simulink model "ACC"  (Simulink 7.5)
settings: Solver=ode45  StartTime=0.0  StopTime=inf  RelTol=1e-3
libraries: CarMaker4SL x24, simulink x2
(part 2 of 2)

== system ACC/CarMaker/Vehicle/CarAndTrailer/Trailer/CreateBus Car.Hitch.FrcTrq ==
  In1 : Inport  OutDataType=sfix(16)  OutScaling=2^0
  Bus Creator7 : BusCreator  Inputs=6
  Demux7 : Demux  Outputs=6
  Car.Hitch.FrcTrq : Outport  OutDataType=sfix(16)  OutScaling=2^0
  wires:
  Demux7/1 -> Bus Creator7/1  "Car Hitch Frc2Car x"
  Demux7/2 -> Bus Creator7/2  "Car Hitch Frc2Car y"
  Demux7/3 -> Bus Creator7/3  "Car Hitch Frc2Car z"
  Demux7/4 -> Bus Creator7/4  "Car Hitch Trq2Car x"
  Demux7/5 -> Bus Creator7/5  "Car Hitch Trq2Car y"
  Demux7/6 -> Bus Creator7/6  "Car Hitch Trq2Car z"
  Bus Creator7/1 -> Car.Hitch.FrcTrq/1
  In1/1 -> Demux7/1

== system ACC/CarMaker/Vehicle/CarAndTrailer/Trailer/CreateBus Vhcl.Motion ==
  In1 : Inport  OutDataType=sfix(16)  OutScaling=2^0
  Demux1 : Demux  Outputs=16
  Mux1 : Mux  Inputs=16
  Out1 : Outport  OutDataType=sfix(16)  OutScaling=2^0
  wires:
  Mux1/1 -> Out1/1
  In1/1 -> Demux1/1
  Demux1/16 -> Mux1/16  "Vhcl YawAcc"
  Demux1/15 -> Mux1/15  "Vhcl YawRate"
  Demux1/14 -> Mux1/14  "Vhcl Yaw"
  Demux1/13 -> Mux1/13  "Vhcl PitchAcc"
  Demux1/12 -> Mux1/12  "Vhcl PitchVel"
  Demux1/11 -> Mux1/11  "Vhcl Pitch"
  Demux1/10 -> Mux1/10  "Vhcl RollAcc"
  Demux1/9 -> Mux1/9  "Vhcl RollVel"
  Demux1/8 -> Mux1/8  "Vhcl Roll"
  Demux1/7 -> Mux1/7  "Vhcl Hitch_Pos z"
  Demux1/6 -> Mux1/6  "Vhcl Hitch_Pos y"
  Demux1/5 -> Mux1/5  "Vhcl Hitch_Pos x"
  Demux1/4 -> Mux1/4  "Vhcl sRoadAero"
  Demux1/3 -> Mux1/3  "Vhcl sRoad"
  Demux1/2 -> Mux1/2  "Vhcl Distance"
  Demux1/1 -> Mux1/1  "Vhcl v"

== system ACC/CarMaker/Vehicle/CarAndTrailer/Trailer/CreateBus Vhcl.PoI ==
  In1 : Inport  OutDataType=sfix(16)  OutScaling=2^0
  Bus Creator3 : BusCreator  Inputs=18
  Demux3 : Demux  Outputs=18
  Out1 : Outport  OutDataType=sfix(16)  OutScaling=2^0
  wires:
  Demux3/1 -> Bus Creator3/1  "Vhcl PoI_Pos x"
  Bus Creator3/1 -> Out1/1
  In1/1 -> Demux3/1
  Demux3/2 -> Bus Creator3/2  "Vhcl PoI_Pos y"
  Demux3/3 -> Bus Creator3/3  "Vhcl PoI_Pos z"
  Demux3/4 -> Bus Creator3/4  "Vhcl PoI_Vel x"
  Demux3/5 -> Bus Creator3/5  "Vhcl PoI_Vel y"
  Demux3/6 -> Bus Creator3/6  "Vhcl PoI_Vel z"
  Demux3/7 -> Bus Creator3/7  "Vhcl PoI_Acc x"
  Demux3/8 -> Bus Creator3/8  "Vhcl PoI_Acc y"
  Demux3/9 -> Bus Creator3/9  "Vhcl PoI_Acc z"
  Demux3/10 -> Bus Creator3/10  "Vhcl PoI_Vel_1 x"
  Demux3/11 -> Bus Creator3/11  "Vhcl PoI_Vel_1 y"
  Demux3/12 -> Bus Creator3/12  "Vhcl PoI_Vel_1 z"
  Demux3/13 -> Bus Creator3/13  "Vhcl PoI_Acc_1 x"
  Demux3/14 -> Bus Creator3/14  "Vhcl PoI_Acc_1 y"
  Demux3/15 -> Bus Creator3/15  "Vhcl PoI_Acc_1 z"
  Demux3/16 -> Bus Creator3/16  "Vhcl PoI_GCS Long"
  Demux3/17 -> Bus Creator3/17  "Vhcl PoI_GCS Lat"
  Demux3/18 -> Bus Creator3/18  "Vhcl PoI_GCS Elev"

== system ACC/CarMaker/Vehicle/CarAndTrailer/Trailer/CreateBus Vhcl.Steering ==
  In1 : Inport  OutDataType=sfix(16)  OutScaling=2^0
  Bus Creator3 : BusCreator
  Demux : Demux
  Out1 : Outport  OutDataType=sfix(16)  OutScaling=2^0
  wires:
  In1/1 -> Demux/1
  Demux/4 -> Bus Creator3/4  "Vhcl Steering Trq"
  Demux/2 -> Bus Creator3/2  "Vhcl Steering AngVel"
  Demux/3 -> Bus Creator3/3  "Vhcl Steering AngAcc"
  Demux/1 -> Bus Creator3/1  "Vhcl Steering Ang"
  Bus Creator3/1 -> Out1/1

== system ACC/CarMaker/Vehicle/CarAndTrailer/Trailer/CreateBus Vhcl.Wheel.FL ==
  In1 : Inport  OutDataType=sfix(16)  OutScaling=2^0
  Bus Creator3 : BusCreator  Inputs=14
  Demux3 : Demux  Outputs=14
  Out1 : Outport  OutDataType=sfix(16)  OutScaling=2^0
  wires:
  Demux3/1 -> Bus Creator3/1  "Vhcl Wheel FL t x"
  Bus Creator3/1 -> Out1/1
  In1/1 -> Demux3/1
  Demux3/2 -> Bus Creator3/2  "Vhcl Wheel FL t y"
  Demux3/3 -> Bus Creator3/3  "Vhcl Wheel FL t z"
  Demux3/4 -> Bus Creator3/4  "Vhcl Wheel FL r_zxy x"
  Demux3/5 -> Bus Creator3/5  "Vhcl Wheel FL r_zxy y"
  Demux3/6 -> Bus Creator3/6  "Vhcl Wheel FL r_zxy z"
  Demux3/7 -> Bus Creator3/7  "Vhcl Wheel FL Fx"
  Demux3/8 -> Bus Creator3/8  "Vhcl Wheel FL Fy"
  Demux3/9 -> Bus Creator3/9  "Vhcl Wheel FL Fz"
  Demux3/10 -> Bus Creator3/10  "Vhcl Wheel FL vBelt"
  Demux3/11 -> Bus Creator3/11  "Vhcl Wheel FL LongSlip"
  Demux3/12 -> Bus Creator3/12  "Vhcl Wheel FL SideSlip"
  Demux3/13 -> Bus Creator3/13  "Vhcl Wheel FL Trq_T2W"
  Demux3/14 -> Bus Creator3/14  "Vhcl Wheel FL Trq_WhlBearing"

== system ACC/CarMaker/Vehicle/CarAndTrailer/Trailer/CreateBus Vhcl.Wheel.FR ==
  In1 : Inport  OutDataType=sfix(16)  OutScaling=2^0
  Bus Creator3 : BusCreator  Inputs=14
  Demux3 : Demux  Outputs=14
  Out1 : Outport  OutDataType=sfix(16)  OutScaling=2^0
  wires:
  Demux3/1 -> Bus Creator3/1  "Vhcl Wheel FR t x"
  Bus Creator3/1 -> Out1/1
  In1/1 -> Demux3/1
  Demux3/2 -> Bus Creator3/2  "Vhcl Wheel FR t y"
  Demux3/3 -> Bus Creator3/3  "Vhcl Wheel FR t z"
  Demux3/4 -> Bus Creator3/4  "Vhcl Wheel FR r_zxy x"
  Demux3/5 -> Bus Creator3/5  "Vhcl Wheel FR r_zxy y"
  Demux3/6 -> Bus Creator3/6  "Vhcl Wheel FR r_zxy z"
  Demux3/7 -> Bus Creator3/7  "Vhcl Wheel FR Fx"
  Demux3/8 -> Bus Creator3/8  "Vhcl Wheel FR Fy"
  Demux3/9 -> Bus Creator3/9  "Vhcl Wheel FR Fz"
  Demux3/10 -> Bus Creator3/10  "Vhcl Wheel FR vBelt"
  Demux3/11 -> Bus Creator3/11  "Vhcl Wheel FR LongSlip"
  Demux3/12 -> Bus Creator3/12  "Vhcl Wheel FR SideSlip"
  Demux3/13 -> Bus Creator3/13  "Vhcl Wheel FR Trq_T2W"
  Demux3/14 -> Bus Creator3/14  "Vhcl Wheel FR Trq_WhlBearing"

== system ACC/CarMaker/Vehicle/CarAndTrailer/Trailer/CreateBus Vhcl.Wheel.RL ==
  In1 : Inport  OutDataType=sfix(16)  OutScaling=2^0
  Bus Creator3 : BusCreator  Inputs=14
  Demux3 : Demux  Outputs=14
  Out1 : Outport  OutDataType=sfix(16)  OutScaling=2^0
  wires:
  Demux3/1 -> Bus Creator3/1  "Vhcl Wheel RL t x"
  Bus Creator3/1 -> Out1/1
  In1/1 -> Demux3/1
  Demux3/2 -> Bus Creator3/2  "Vhcl Wheel RL t y"
  Demux3/3 -> Bus Creator3/3  "Vhcl Wheel RL t z"
  Demux3/4 -> Bus Creator3/4  "Vhcl Wheel RL r_zxy x"
  Demux3/5 -> Bus Creator3/5  "Vhcl Wheel RL r_zxy y"
  Demux3/6 -> Bus Creator3/6  "Vhcl Wheel RL r_zxy z"
  Demux3/7 -> Bus Creator3/7  "Vhcl Wheel RL Fx"
  Demux3/8 -> Bus Creator3/8  "Vhcl Wheel RL Fy"
  Demux3/9 -> Bus Creator3/9  "Vhcl Wheel RL Fz"
  Demux3/10 -> Bus Creator3/10  "Vhcl Wheel RL vBelt"
  Demux3/11 -> Bus Creator3/11  "Vhcl Wheel RL LongSlip"
  Demux3/12 -> Bus Creator3/12  "Vhcl Wheel RL SideSlip"
  Demux3/13 -> Bus Creator3/13  "Vhcl Wheel RL Trq_T2W"
  Demux3/14 -> Bus Creator3/14  "Vhcl Wheel RL Trq_WhlBearing"

== system ACC/CarMaker/Vehicle/CarAndTrailer/Trailer/CreateBus Vhcl.Wheel.RR ==
  In1 : Inport  OutDataType=sfix(16)  OutScaling=2^0
  Bus Creator3 : BusCreator  Inputs=14
  Demux3 : Demux  Outputs=14
  Out1 : Outport  OutDataType=sfix(16)  OutScaling=2^0
  wires:
  Demux3/1 -> Bus Creator3/1  "Vhcl Wheel RR t x"
  Bus Creator3/1 -> Out1/1
  In1/1 -> Demux3/1
  Demux3/2 -> Bus Creator3/2  "Vhcl Wheel RR t y"
  Demux3/3 -> Bus Creator3/3  "Vhcl Wheel RR t z"
  Demux3/4 -> Bus Creator3/4  "Vhcl Wheel RR r_zxy x"
  Demux3/5 -> Bus Creator3/5  "Vhcl Wheel RR r_zxy y"
  Demux3/6 -> Bus Creator3/6  "Vhcl Wheel RR r_zxy z"
  Demux3/7 -> Bus Creator3/7  "Vhcl Wheel RR Fx"
  Demux3/8 -> Bus Creator3/8  "Vhcl Wheel RR Fy"
  Demux3/9 -> Bus Creator3/9  "Vhcl Wheel RR Fz"
  Demux3/10 -> Bus Creator3/10  "Vhcl Wheel RR vBelt"
  Demux3/11 -> Bus Creator3/11  "Vhcl Wheel RR LongSlip"
  Demux3/12 -> Bus Creator3/12  "Vhcl Wheel RR SideSlip"
  Demux3/13 -> Bus Creator3/13  "Vhcl Wheel RR Trq_T2W"
  Demux3/14 -> Bus Creator3/14  "Vhcl Wheel RR Trq_WhlBearing"

== system ACC/CarMaker/VehicleControl/ACC/ACC ECU/ACC Control ==
  ACC enabled : Inport  OutDataType=sfix(16)  OutScaling=2^0
  Target Dtct : Inport  Port=2  OutDataType=sfix(16)  OutScaling=2^0
  Target.ds : Inport  Port=3  OutDataType=sfix(16)  OutScaling=2^0
  Target.dv : Inport  Port=4  OutDataType=sfix(16)  OutScaling=2^0
  Desired time gap : Inport  Port=5  OutDataType=sfix(16)  OutScaling=2^0
  Desired speed : Inport  Port=6  OutDataType=sfix(16)  OutScaling=2^0
  Desired Distance Calculation with time gap : Subsystem  TreatAsAtomicUnit=on
  Distance Control Algorithm : Subsystem  TreatAsAtomicUnit=on
  Logical Operator : Logic  AllPortsSameDT=off
  Speed Control Algorithm : Subsystem  TreatAsAtomicUnit=on
  Target detected : simulink/Logic and Bit Operations/Compare To Zero  SystemSampleTime=-1  relop=>  LogicOutDataTypeMode=uint8  ZeroCross=off
  Zero Ax : Constant  Value=0  OutDataType=sfix(16)  OutScaling=2^0
  desired ax : Switch  Threshold=1  SaturateOnIntegerOverflow=on
  desired or zero : Switch  Threshold=1  SaturateOnIntegerOverflow=on
  Desired Ax : Outport  OutDataType=sfix(16)  OutScaling=2^0
  wires:
  Zero Ax/1 -> desired or zero/3
  desired ax/1 -> desired or zero/1
  desired or zero/1 -> Desired Ax/1
  Logical Operator/1 -> Desired Distance Calculation with time gap/Enable
  ACC enabled/1 -> desired or zero/2, Logical Operator/1
  Speed Control Algorithm/1(ax speed control) -> Distance Control Algorithm/4(ax speed control), desired ax/3
  Desired speed/1 -> Speed Control Algorithm/1(desire speed[m/s])
  Desired time gap/1 -> Desired Distance Calculation with time gap/2(desired time gap)
  Desired Distance Calculation with time gap/1(desired distance) -> Distance Control Algorithm/3(desired distance[m])
  Target detected/1 -> Logical Operator/2, desired ax/2
  Distance Control Algorithm/1("  limited ax") -> desired ax/1
  Target Dtct/1 -> Target detected/1
  Target.ds/1 -> Distance Control Algorithm/1(Target.ds[m])
  Target.dv/1 -> Desired Distance Calculation with time gap/1(Target.dv), Distance Control Algorithm/2(Target.dv[m/s])

== system ACC/CarMaker/VehicleControl/ACC/ACC ECU/ACC User Input ==
  ACC Active ACC/Actual Speed : Switch  Threshold=1  SaturateOnIntegerOverflow=on
  Constant : Constant  OutDataType=sfix(16)  OutScaling=2^0
  Init Desired time gap quantity : Subsystem  TreatAsAtomicUnit=on
  Is ACC enabled : CarMaker4SL/Read CM Dict  xname=AccelCtrl.ACC.IsActive  xsync=off
  Memory : Memory
  Read Car.v[m/s] : CarMaker4SL/Read CM Dict  xname=Car.v  xsync=off
  Read User desired speed : CarMaker4SL/Read CM Dict  xname=AccelCtrl.ACC.DesiredSpd  xsync=off
  Read User desired time gap : CarMaker4SL/Read CM Dict  xname=AccelCtrl.ACC.DesiredTGap  xsync=off
  Read init desired time gap from Inf : CarMaker4SL/Read CM Parameter  xfile=Vehicle  xkey=AccelCtrl.ACC.DesrTGap  xnout=1  xdefaults=1.8  xmuxed=off
  Write desired speed : CarMaker4SL/Write CM Dict  xname=AccelCtrl.ACC.DesiredSpd  xsync=off
  ACC enabled : Outport  OutDataType=sfix(16)  OutScaling=2^0
  Desired time gap[s] : Outport  Port=2  OutDataType=sfix(16)  OutScaling=2^0
  Desired speed[m/s] : Outport  Port=3  OutDataType=sfix(16)  OutScaling=2^0
  wires:
  Read init desired time gap from Inf/1 -> Init Desired time gap quantity/1("Init desired time gap ")
  Memory/1 -> Init Desired time gap quantity/Trigger
  Constant/1 -> Memory/1
  Read User desired time gap/1 -> Desired time gap[s]/1
  ACC Active ACC/Actual Speed/1 -> Write desired speed/1, Desired speed[m/s]/1
  Read Car.v[m/s]/1 -> ACC Active ACC/Actual Speed/3
  Read User desired speed/1 -> ACC Active ACC/Actual Speed/1
  Is ACC enabled/1 -> ACC Active ACC/Actual Speed/2, ACC enabled/1

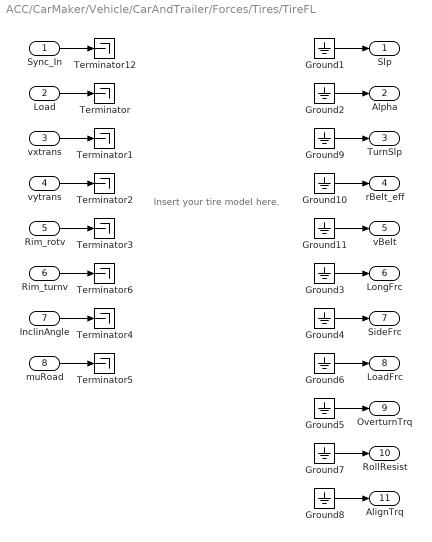
== system ACC/CarMaker/Vehicle/CarAndTrailer/Forces/Tires/TireFL ==
  note: Insert your tire model here.
  Sync_In : Inport  OutDataType=sfix(16)  OutScaling=2^0
  Load : Inport  Port=2  OutDataType=sfix(16)  OutScaling=2^0
  vxtrans : Inport  Port=3  OutDataType=sfix(16)  OutScaling=2^0
  vytrans : Inport  Port=4  OutDataType=sfix(16)  OutScaling=2^0
  Rim_rotv : Inport  Port=5  OutDataType=sfix(16)  OutScaling=2^0
  Rim_turnv : Inport  Port=6  OutDataType=sfix(16)  OutScaling=2^0
  InclinAngle : Inport  Port=7  OutDataType=sfix(16)  OutScaling=2^0
  muRoad : Inport  Port=8  OutDataType=sfix(16)  OutScaling=2^0
  Ground{1..11} (11 alike) : Ground
  Terminator{,1..6,12} (8 alike) : Terminator
  Slp : Outport  OutDataType=sfix(16)  OutScaling=2^0
  Alpha : Outport  Port=2  OutDataType=sfix(16)  OutScaling=2^0
  TurnSlp : Outport  Port=3  OutDataType=sfix(16)  OutScaling=2^0
  rBelt_eff : Outport  Port=4  OutDataType=sfix(16)  OutScaling=2^0
  vBelt : Outport  Port=5  OutDataType=sfix(16)  OutScaling=2^0
  LongFrc : Outport  Port=6  OutDataType=sfix(16)  OutScaling=2^0
  SideFrc : Outport  Port=7  OutDataType=sfix(16)  OutScaling=2^0
  LoadFrc : Outport  Port=8  OutDataType=sfix(16)  OutScaling=2^0
  OverturnTrq : Outport  Port=9  OutDataType=sfix(16)  OutScaling=2^0
  RollResist : Outport  Port=10  OutDataType=sfix(16)  OutScaling=2^0
  AlignTrq : Outport  Port=11  OutDataType=sfix(16)  OutScaling=2^0
  wires:
  Ground8/1 -> AlignTrq/1
  Ground7/1 -> RollResist/1
  Ground6/1 -> LoadFrc/1
  Ground1/1 -> Slp/1
  Load/1 -> Terminator/1
  muRoad/1 -> Terminator5/1
  InclinAngle/1 -> Terminator4/1
  Rim_rotv/1 -> Terminator3/1
  vytrans/1 -> Terminator2/1
  vxtrans/1 -> Terminator1/1
  Ground5/1 -> OverturnTrq/1
  Ground4/1 -> SideFrc/1
  Ground3/1 -> LongFrc/1
  Ground2/1 -> Alpha/1
  Sync_In/1 -> Terminator12/1
  Rim_turnv/1 -> Terminator6/1
  Ground9/1 -> TurnSlp/1
  Ground10/1 -> rBelt_eff/1
  Ground11/1 -> vBelt/1

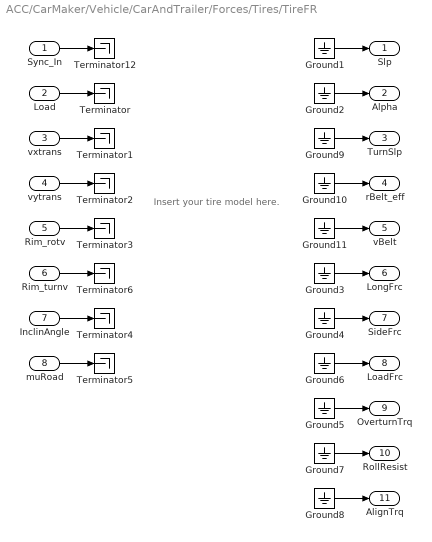
== system ACC/CarMaker/Vehicle/CarAndTrailer/Forces/Tires/TireFR ==
  note: Insert your tire model here.
  Sync_In : Inport  OutDataType=sfix(16)  OutScaling=2^0
  Load : Inport  Port=2  OutDataType=sfix(16)  OutScaling=2^0
  vxtrans : Inport  Port=3  OutDataType=sfix(16)  OutScaling=2^0
  vytrans : Inport  Port=4  OutDataType=sfix(16)  OutScaling=2^0
  Rim_rotv : Inport  Port=5  OutDataType=sfix(16)  OutScaling=2^0
  Rim_turnv : Inport  Port=6  OutDataType=sfix(16)  OutScaling=2^0
  InclinAngle : Inport  Port=7  OutDataType=sfix(16)  OutScaling=2^0
  muRoad : Inport  Port=8  OutDataType=sfix(16)  OutScaling=2^0
  Ground{1..11} (11 alike) : Ground
  Terminator{,1..6,12} (8 alike) : Terminator
  Slp : Outport  OutDataType=sfix(16)  OutScaling=2^0
  Alpha : Outport  Port=2  OutDataType=sfix(16)  OutScaling=2^0
  TurnSlp : Outport  Port=3  OutDataType=sfix(16)  OutScaling=2^0
  rBelt_eff : Outport  Port=4  OutDataType=sfix(16)  OutScaling=2^0
  vBelt : Outport  Port=5  OutDataType=sfix(16)  OutScaling=2^0
  LongFrc : Outport  Port=6  OutDataType=sfix(16)  OutScaling=2^0
  SideFrc : Outport  Port=7  OutDataType=sfix(16)  OutScaling=2^0
  LoadFrc : Outport  Port=8  OutDataType=sfix(16)  OutScaling=2^0
  OverturnTrq : Outport  Port=9  OutDataType=sfix(16)  OutScaling=2^0
  RollResist : Outport  Port=10  OutDataType=sfix(16)  OutScaling=2^0
  AlignTrq : Outport  Port=11  OutDataType=sfix(16)  OutScaling=2^0
  wires:
  Ground8/1 -> AlignTrq/1
  Ground7/1 -> RollResist/1
  Ground6/1 -> LoadFrc/1
  Ground1/1 -> Slp/1
  Load/1 -> Terminator/1
  muRoad/1 -> Terminator5/1
  InclinAngle/1 -> Terminator4/1
  Rim_rotv/1 -> Terminator3/1
  vytrans/1 -> Terminator2/1
  vxtrans/1 -> Terminator1/1
  Ground5/1 -> OverturnTrq/1
  Ground4/1 -> SideFrc/1
  Ground3/1 -> LongFrc/1
  Ground2/1 -> Alpha/1
  Sync_In/1 -> Terminator12/1
  Rim_turnv/1 -> Terminator6/1
  Ground9/1 -> TurnSlp/1
  Ground10/1 -> rBelt_eff/1
  Ground11/1 -> vBelt/1

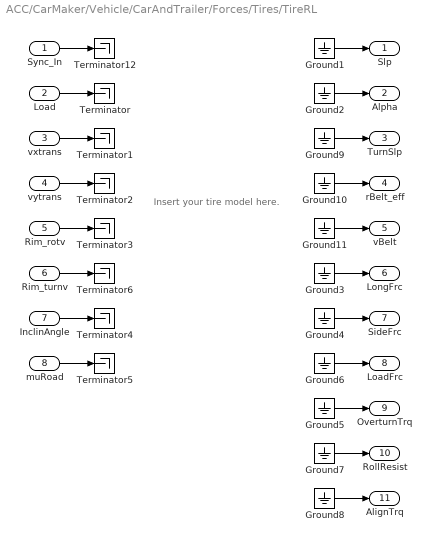
== system ACC/CarMaker/Vehicle/CarAndTrailer/Forces/Tires/TireRL ==
  note: Insert your tire model here.
  Sync_In : Inport  OutDataType=sfix(16)  OutScaling=2^0
  Load : Inport  Port=2  OutDataType=sfix(16)  OutScaling=2^0
  vxtrans : Inport  Port=3  OutDataType=sfix(16)  OutScaling=2^0
  vytrans : Inport  Port=4  OutDataType=sfix(16)  OutScaling=2^0
  Rim_rotv : Inport  Port=5  OutDataType=sfix(16)  OutScaling=2^0
  Rim_turnv : Inport  Port=6  OutDataType=sfix(16)  OutScaling=2^0
  InclinAngle : Inport  Port=7  OutDataType=sfix(16)  OutScaling=2^0
  muRoad : Inport  Port=8  OutDataType=sfix(16)  OutScaling=2^0
  Ground{1..11} (11 alike) : Ground
  Terminator{,1..6,12} (8 alike) : Terminator
  Slp : Outport  OutDataType=sfix(16)  OutScaling=2^0
  Alpha : Outport  Port=2  OutDataType=sfix(16)  OutScaling=2^0
  TurnSlp : Outport  Port=3  OutDataType=sfix(16)  OutScaling=2^0
  rBelt_eff : Outport  Port=4  OutDataType=sfix(16)  OutScaling=2^0
  vBelt : Outport  Port=5  OutDataType=sfix(16)  OutScaling=2^0
  LongFrc : Outport  Port=6  OutDataType=sfix(16)  OutScaling=2^0
  SideFrc : Outport  Port=7  OutDataType=sfix(16)  OutScaling=2^0
  LoadFrc : Outport  Port=8  OutDataType=sfix(16)  OutScaling=2^0
  OverturnTrq : Outport  Port=9  OutDataType=sfix(16)  OutScaling=2^0
  RollResist : Outport  Port=10  OutDataType=sfix(16)  OutScaling=2^0
  AlignTrq : Outport  Port=11  OutDataType=sfix(16)  OutScaling=2^0
  wires:
  Ground8/1 -> AlignTrq/1
  Ground7/1 -> RollResist/1
  Ground6/1 -> LoadFrc/1
  Ground1/1 -> Slp/1
  Load/1 -> Terminator/1
  muRoad/1 -> Terminator5/1
  InclinAngle/1 -> Terminator4/1
  Rim_rotv/1 -> Terminator3/1
  vytrans/1 -> Terminator2/1
  vxtrans/1 -> Terminator1/1
  Ground5/1 -> OverturnTrq/1
  Ground4/1 -> SideFrc/1
  Ground3/1 -> LongFrc/1
  Ground2/1 -> Alpha/1
  Sync_In/1 -> Terminator12/1
  Rim_turnv/1 -> Terminator6/1
  Ground9/1 -> TurnSlp/1
  Ground10/1 -> rBelt_eff/1
  Ground11/1 -> vBelt/1

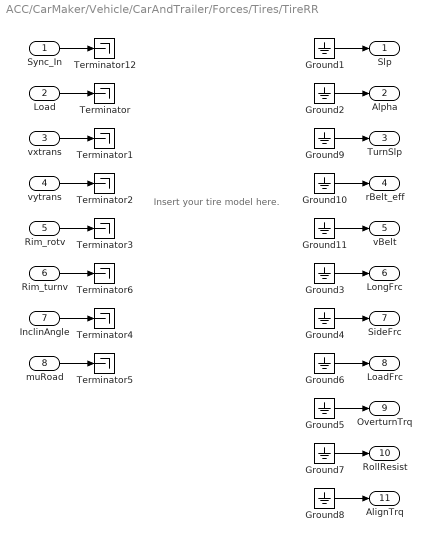
== system ACC/CarMaker/Vehicle/CarAndTrailer/Forces/Tires/TireRR ==
  note: Insert your tire model here.
  Sync_In : Inport  OutDataType=sfix(16)  OutScaling=2^0
  Load : Inport  Port=2  OutDataType=sfix(16)  OutScaling=2^0
  vxtrans : Inport  Port=3  OutDataType=sfix(16)  OutScaling=2^0
  vytrans : Inport  Port=4  OutDataType=sfix(16)  OutScaling=2^0
  Rim_rotv : Inport  Port=5  OutDataType=sfix(16)  OutScaling=2^0
  Rim_turnv : Inport  Port=6  OutDataType=sfix(16)  OutScaling=2^0
  InclinAngle : Inport  Port=7  OutDataType=sfix(16)  OutScaling=2^0
  muRoad : Inport  Port=8  OutDataType=sfix(16)  OutScaling=2^0
  Ground{1..11} (11 alike) : Ground
  Terminator{,1..6,12} (8 alike) : Terminator
  Slp : Outport  OutDataType=sfix(16)  OutScaling=2^0
  Alpha : Outport  Port=2  OutDataType=sfix(16)  OutScaling=2^0
  TurnSlp : Outport  Port=3  OutDataType=sfix(16)  OutScaling=2^0
  rBelt_eff : Outport  Port=4  OutDataType=sfix(16)  OutScaling=2^0
  vBelt : Outport  Port=5  OutDataType=sfix(16)  OutScaling=2^0
  LongFrc : Outport  Port=6  OutDataType=sfix(16)  OutScaling=2^0
  SideFrc : Outport  Port=7  OutDataType=sfix(16)  OutScaling=2^0
  LoadFrc : Outport  Port=8  OutDataType=sfix(16)  OutScaling=2^0
  OverturnTrq : Outport  Port=9  OutDataType=sfix(16)  OutScaling=2^0
  RollResist : Outport  Port=10  OutDataType=sfix(16)  OutScaling=2^0
  AlignTrq : Outport  Port=11  OutDataType=sfix(16)  OutScaling=2^0
  wires:
  Ground8/1 -> AlignTrq/1
  Ground7/1 -> RollResist/1
  Ground6/1 -> LoadFrc/1
  Ground1/1 -> Slp/1
  Load/1 -> Terminator/1
  muRoad/1 -> Terminator5/1
  InclinAngle/1 -> Terminator4/1
  Rim_rotv/1 -> Terminator3/1
  vytrans/1 -> Terminator2/1
  vxtrans/1 -> Terminator1/1
  Ground5/1 -> OverturnTrq/1
  Ground4/1 -> SideFrc/1
  Ground3/1 -> LongFrc/1
  Ground2/1 -> Alpha/1
  Sync_In/1 -> Terminator12/1
  Rim_turnv/1 -> Terminator6/1
  Ground9/1 -> TurnSlp/1
  Ground10/1 -> rBelt_eff/1
  Ground11/1 -> vBelt/1

== system ACC/CarMaker/VehicleControl/ACC/ACC ECU/ACC Control/Desired Distance Calculation with time gap ==
  Target.dv : Inport  OutDataType=sfix(16)  OutScaling=2^0
  desired time gap : Inport  Port=2  OutDataType=sfix(16)  OutScaling=2^0
  Enable : EnablePort
  Add : Sum  OutDataType=sfix(16)  OutScaling=2^-10  SaturateOnIntegerOverflow=on  OutDataTypeStr=Inherit: Same as first input
  Initial min distance : CarMaker4SL/Read CM Parameter  xfile=Vehicle  xkey=AccelCtrl.ACC.DistMin  xnout=1  xdefaults=20  xmuxed=off
  MinMax : MinMax  Function=max  Inputs=2  OutDataType=sfix(16)  OutScaling=2^0  SaturateOnIntegerOverflow=on  InputSameDT=on
  Product : Product  OutDataType=sfix(16)  OutScaling=2^0  SaturateOnIntegerOverflow=on  OutDataTypeStr=Inherit: Same as first input
  Read Car.v[m/s] : CarMaker4SL/Read CM Dict  xname=Car.v  xsync=off
  Write desired distance : CarMaker4SL/Write CM Dict  xname=AccelCtrl.ACC.DesiredDist  xsync=off
  desired distance : Outport  OutDataType=sfix(16)  OutScaling=2^0  InitialOutput=0
  wires:
  Initial min distance/1 -> MinMax/2
  MinMax/1 -> Write desired distance/1, desired distance/1
  Target.dv/1 -> Add/1
  desired time gap/1 -> Product/1
  Add/1 -> Product/2
  Product/1 -> MinMax/1
  Read Car.v[m/s]/1 -> Add/2

== system ACC/CarMaker/VehicleControl/ACC/ACC ECU/ACC Control/Distance Control Algorithm ==
  Target.ds[m] : Inport  OutDataType=sfix(16)  OutScaling=2^0
  Target.dv[m/s] : Inport  Port=2  OutDataType=sfix(16)  OutScaling=2^0
  desired distance[m] : Inport  Port=3  OutDataType=sfix(16)  OutScaling=2^0
  ax speed control : Inport  Port=4  OutDataType=sfix(16)  OutScaling=2^0
  -2.5<=ax<=1 : Saturate  UpperLimit=1  LowerLimit=-2.5
  desired ax : Subsystem
  "  limited ax" : Outport  OutDataType=sfix(16)  OutScaling=2^0  InitialOutput=0
  wires:
  desired ax/1(desired ax) -> -2.5<=ax<=1/1
  -2.5<=ax<=1/1 -> "  limited ax"/1
  Target.ds[m]/1 -> desired ax/1(Target.ds[m])
  Target.dv[m/s]/1 -> desired ax/2(Target.dv[m/s])
  desired distance[m]/1 -> desired ax/3(desired distance[m])
  ax speed control/1 -> desired ax/4(ax speed control)

== system ACC/CarMaker/VehicleControl/ACC/ACC ECU/ACC Control/Speed Control Algorithm ==
  desire speed[m/s] : Inport  OutDataType=sfix(16)  OutScaling=2^0
  -0.35<=ax<=1 : Saturate  UpperLimit=1  LowerLimit=-0.35
  desired ax : Subsystem
  ax speed control : Outport  OutDataType=sfix(16)  OutScaling=2^0  InitialOutput=0
  wires:
  -0.35<=ax<=1/1 -> ax speed control/1
  desired ax/1(desired ax) -> -0.35<=ax<=1/1
  desire speed[m/s]/1 -> desired ax/1(desire speed[m/s])

== system ACC/CarMaker/VehicleControl/ACC/ACC ECU/ACC User Input/Init Desired time gap quantity ==
  "Init desired time gap " : Inport  OutDataType=sfix(16)  OutScaling=2^0
  Trigger : TriggerPort
  Write init time gap : CarMaker4SL/Write CM Dict  xname=AccelCtrl.ACC.DesiredTGap  xsync=off
  wires:
  "Init desired time gap "/1 -> Write init time gap/1

== system ACC/CarMaker/VehicleControl/ACC/ACC ECU/ACC Control/Distance Control Algorithm/desired ax ==
  note: delta_ds
  note: desired ax = (target.ds-desired.distance)/(kd)+target.dv/kv
  Target.ds[m] : Inport  OutDataType=sfix(16)  OutScaling=2^0
  Target.dv[m/s] : Inport  Port=2  OutDataType=sfix(16)  OutScaling=2^0
  desired distance[m] : Inport  Port=3  OutDataType=sfix(16)  OutScaling=2^0
  ax speed control : Inport  Port=4  OutDataType=sfix(16)  OutScaling=2^0
  Add : Sum  OutDataType=sfix(16)  OutScaling=2^-10  SaturateOnIntegerOverflow=on  OutDataTypeStr=Inherit: Same as first input
  Divide : Product  Inputs=*/  OutDataType=sfix(16)  OutScaling=2^-10  SaturateOnIntegerOverflow=on  OutDataTypeStr=Inherit: Same as first input
  Divide1 : Product  Inputs=*/  OutDataType=sfix(16)  OutScaling=2^-10  SaturateOnIntegerOverflow=on  OutDataTypeStr=Inherit: Same as first input
  Initial distctrl.kd : CarMaker4SL/Read CM Parameter  xfile=Vehicle  xkey=AccelCtrl.ACC.DistCtrl.kd  xnout=1  xdefaults=36  xmuxed=off
  Initial distctrl.kv : CarMaker4SL/Read CM Parameter  xfile=Vehicle  xkey=AccelCtrl.ACC.DistCtrl.kv  xnout=1  xdefaults=2  xmuxed=off
  MinMax : MinMax  Inputs=2  OutDataType=sfix(16)  OutScaling=2^0  SaturateOnIntegerOverflow=on  InputSameDT=on
  Subtract : Sum  Inputs=+-  OutDataType=sfix(16)  OutScaling=2^-10  SaturateOnIntegerOverflow=on  OutDataTypeStr=Inherit: Same as first input
  desired ax : Outport  OutDataType=sfix(16)  OutScaling=2^0
  wires:
  Initial distctrl.kv/1 -> Divide1/2
  Initial distctrl.kd/1 -> Divide/2
  Target.dv[m/s]/1 -> Divide1/1
  Target.ds[m]/1 -> Subtract/1
  desired distance[m]/1 -> Subtract/2
  Subtract/1 -> Divide/1
  Divide/1 -> Add/1
  Divide1/1 -> Add/2
  Add/1 -> MinMax/1
  ax speed control/1 -> MinMax/2
  MinMax/1 -> desired ax/1

== system ACC/CarMaker/VehicleControl/ACC/ACC ECU/ACC Control/Speed Control Algorithm/desired ax ==
  desire speed[m/s] : Inport  OutDataType=sfix(16)  OutScaling=2^0
  Divide : Product  Inputs=*/  OutDataType=sfix(16)  OutScaling=2^-10  SaturateOnIntegerOverflow=on  OutDataTypeStr=Inherit: Same as first input
  Initial spdctrl.kv : CarMaker4SL/Read CM Parameter  xfile=Vehicle  xkey=AccelCtrl.ACC.SpdCtrl.kv  xnout=1  xdefaults=13  xmuxed=off
  Read Car.v[m/s] : CarMaker4SL/Read CM Dict  xname=Car.v  xsync=off
  Sum : Sum  Inputs=|+-  OutDataType=sfix(16)  OutScaling=2^0  SaturateOnIntegerOverflow=on  OutDataTypeStr=Inherit: Same as first input
  desired ax : Outport  OutDataType=sfix(16)  OutScaling=2^0
  wires:
  Initial spdctrl.kv/1 -> Divide/2
  Sum/1 -> Divide/1
  Read Car.v[m/s]/1 -> Sum/2
  desire speed[m/s]/1 -> Sum/1
  Divide/1 -> desired ax/1
